simulink model "Power_windows"  (R2017b)
settings: Solver=VariableStepAuto  StartTime=0.0  StopTime=30  RelTol=1e-3
undefined symbols (not defined in the file): sigbuilder_block
libraries: simulink x1
settings Model: PauseTimes=10  SnapshotBufferSize=1  SnapshotInterval=1  Creator=ECoDe_user13  LastModifiedBy=ECoDe_user11
settings DebuggingCC: SignalInfNanChecking=error  UniqueDataStoreMsg=error  StrictBusMsg=ErrorOnBusTreatedAsVector
settings ConfigComp: CovEnable=on  RecordCoverage=on  CovMetricSettings=dcmwe  CovModelRefEnable=on

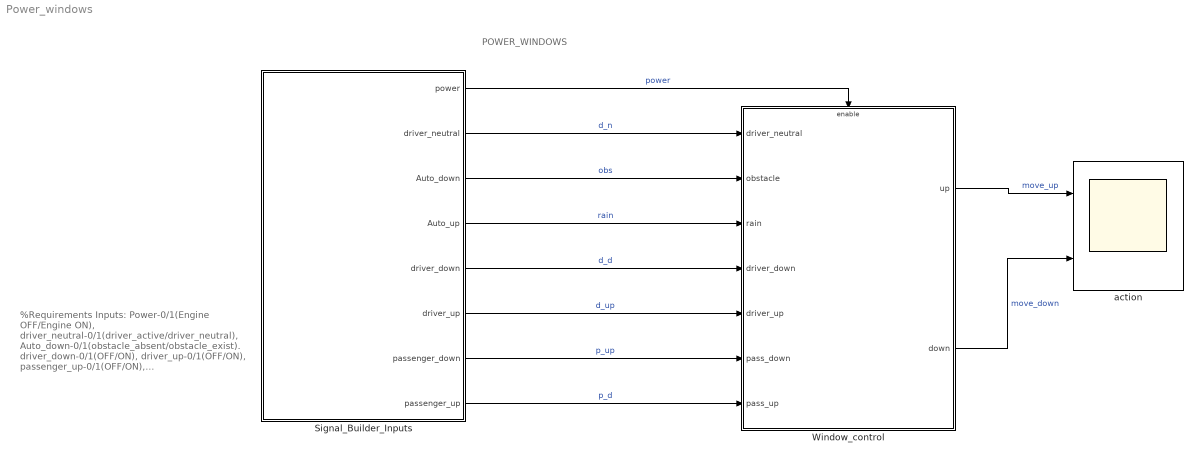
== system Power_windows ==
  note: POWER_WINDOWS
  note: %Requirements
      | Inputs:
      | Power-0/1(Engine OFF/Engine ON),
      | driver_neutral-0/1(driver_active/driver_neutral),
      | Auto_down-0/1(obstacle_absent/obstacle_exist).
      | driver_down-0/1(OFF/ON),
      | driver_up-0/1(OFF/ON),
      | passenger_up-0/1(OFF/ON),
      | passenger_down-0/1(OFF/ON),
      | Outputs:
      | Move_up-0/1(Either_neutral/UP),
      | Move_down-0/1(Either_neutral/Down.
  Signal_Builder_Inputs : Subsystem  Tag=STV Subsys  LoadFcn=sigbuilder_block('load',[3 150.75 550.5 369 ]);  StartFcn=sigbuilder_block('start');  StopFcn=sigbuilder_block('stop');  ClipboardFcn=sigbuilder_block('clipboard');  mask(Sigbuilder block){tuvar=[0:10]}
      mask help: Simulink:masks:SigbuilderBlock_MD
      mask init:
      | if ~strcmp(get_param(bdroot(gcbh),'SimulationStatus'),'stopped') tuvar = sigbuilder_block('maskInit'); end
      settings: CopyFcn=sigbuilder_block('copy');  DeleteFcn=sigbuilder_block('delete');  ModelCloseFcn=sigbuilder_block('modelClose');  PreSaveFcn=sigbuilder_block('preSave');  PauseFcn=sigbuilder_block('pause');  ContinueFcn=sigbuilder_block('continue');  NameChangeFcn=sigbuilder_block('namechange');  OpenFcn=sigbuilder_block('open',[3 150.75 550.5 369 ]);  CloseFcn=sigbuilder_block('close');
      mask Display: plot(0, 0, 100, 100,[2, 2, 32, 32, 2], [68, 8, 8, 68, 68],[32, 2], [38, 38], [32, 19, 2],[53, 60, 44], [32, 17, 17, 2],[16, 16, 31, 31]);txt = getActiveGroup(gcbh);text(2, 100, txt,'verticalAlignment', 'top');
  Window_control : Subsystem
  action : Scope  NumInputPorts=2
  wires:
  Signal_Builder_Inputs/1(power) -> Window_control/Enable  "power"
  Signal_Builder_Inputs/3(Auto_down) -> Window_control/2(obstacle)  "obs"
  Signal_Builder_Inputs/4(Auto_up) -> Window_control/3(rain)  "rain"
  Signal_Builder_Inputs/5(driver_down) -> Window_control/4(driver_down)  "d_d"
  Signal_Builder_Inputs/6(driver_up) -> Window_control/5(driver_up)  "d_up"
  Signal_Builder_Inputs/7(passenger_down) -> Window_control/6(pass_down)  "p_up"
  Signal_Builder_Inputs/8(passenger_up) -> Window_control/7(pass_up)  "p_d"
  Window_control/1(up) -> action/1  "move_up"
  Window_control/2(down) -> action/2  "move_down"
  Signal_Builder_Inputs/2(driver_neutral) -> Window_control/1(driver_neutral)  "d_n"

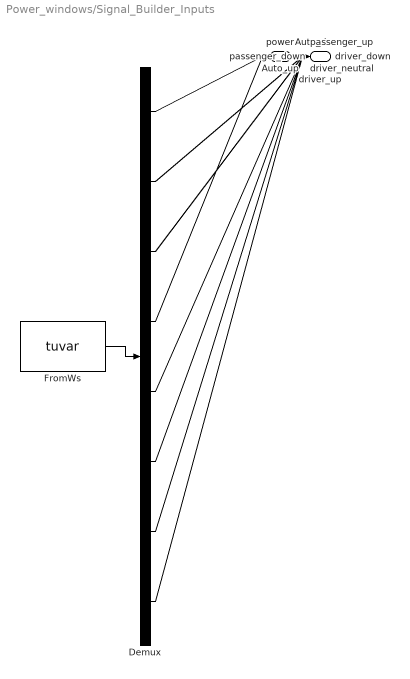
== system Power_windows/Signal_Builder_Inputs ==
  Demux : Demux  Tag=STV Demux  Outputs=8
  FromWs : FromWorkspace  Tag=STV FromWs  VariableName=tuvar  SampleTime=0
      SigBuilderData=|
      | common.afterFinalStr = 'Extrapolate'
      | common.sampleTime = 0
      | dataSet.timeRange = [0 28]
      | dataSet.name = 'Inputs'
      | sbobj.Name = 'Signal Builder'
      | sbobj.Groups.Name = 'Inputs'
      | sbobj.Groups.Signals(1).Name = 'power'
      | sbobj.Groups.Signals(1).XData = [0 1 2 3 4 5 6 7 8 9 10 11 12 13 14 15 16 17 18 19 20 20 21 21 22 22 23 24 25 26 26 27 28]
      | sbobj.Groups.Signals(1).YData = [1 1 1 1 1 1 1 1 1 1 1 1 1 1 1 1 1 1 1 1 1 0 0 1 1 0 0 0 0 0 1 1 1]
      | sbobj.Groups.Signals(2).Name = 'driver_neutral'
      | sbobj.Groups.Signals(2).XData = [0 1 1 2 3 3 4 5 5 6 6 7 8 8 9 10 10 11 11 12 13 13 14 15 15 16 16 17 18 18 19 20 21 22 22 23 23 24 25 26 27 28]
      | sbobj.Groups.Signals(2).YData = [0 0 1 1 1 0 0 0 1 1 0 0 0 1 1 1 0 0 1 1 1 0 0 0 1 1 0 0 0 1 1 1 1 1 0 0 1 1 1 1 1 1]
      | sbobj.Groups.Signals(3).Name = 'Auto_down'
      | sbobj.Groups.Signals(3).XData = [0 1 2 3 4 5 5 6 6 7 8 9 10 11 12 13 14 15 15 16 16 17 18 19 20 21 21 22 22 23 24 25 26 26 27 28]
      | sbobj.Groups.Signals(3).YData = [0 0 0 0 0 0 1 1 0 0 0 0 0 0 0 0 0 0 1 1 0 0 0 0 0 0 1 1 0 0 0 0 0 1 1 1]
      | sbobj.Groups.Signals(4).Name = 'Auto_up'
      | sbobj.Groups.Signals(4).XData = [0 1 2 2 3 3 4 5 6 7 7 8 8 9 9 10 10 11 12 12 13 13 14 15 16 17 17 18 18 19 19 20 20 21 21 22 23 23 24 24 25 25 26 26 27 28]
      | sbobj.Groups.Signals(4).YData = [0 0 0 1 1 0 0 0 0 0 1 1 0 0 1 1 0 0 0 1 1 0 0 0 0 0 1 1 0 0 1 1 0 0 1 1 1 0 0 1 1 0 0 1 1 1]
      | sbobj.Groups.Signals(5).Name = 'driver_down'
      | sbobj.Groups.Signals(5).XData = [0 1 1 2 3 3 4 4 5 6 6 7 8 8 9 10 10 11 11 12 13 13 14 14 15 16 16 17 18 18 19 20 21 22 22 23 23 24 25 25 26 27 28]
      | sbobj.Groups.Signals(5).YData = [1 1 0 0 0 1 1 0 0 0 1 1 1 0 0 0 1 1 0 0 0 1 1 0 0 0 1 1 1 0 0 0 0 0 1 1 0 0 0 1 1 1 1]
      | sbobj.Groups.Signals(6).Name = 'driver_up'
      | sbobj.Groups.Signals(6).XData = [0 1 2 3 4 4 5 5 6 7 8 9 10 11 12 13 14 14 15 15 16 17 18 19 20 21 21 22 22 23 24 25 26 26 27 27 28]
      | sbobj.Groups.Signals(6).YData = [0 0 0 0 0 1 1 0 0 0 0 0 0 0 0 0 0 1 1 0 0 0 0 0 0 0 1 1 0 0 0 0 0 1 1 0 0]
      | sbobj.Groups.Signals(7).Name = 'passenger_down'
      | sbobj.Groups.Signals(7).XData = [0 1 2 3 4 4 5 5 6 7 7 8 9 10 10 11 11 12 12 13 14 14 15 15 16 17 17 18 19 20 20 21 21 22 23 24 25 25 26 26 27 28]
      | sbobj.Groups.Signals(7).YData = [0 0 0 0 0 1 1 0 0 0 1 1 1 1 0 0 1 1 0 0 0 1 1 0 0 0 1 1 1 1 0 0 1 1 1 1 1 0 0 1 1 1]
      | sbobj.Groups.Signals(8).Name = 'passenger_up'
      | sbobj.Groups.Signals(8).XData = [0 1 1 2 2 3 3 4 4 5 5 6 7 7 8 9 10 11 12 13 13 14 14 15 15 16 17 17 18 19 20 21 21 22 22 23 24 25 26 26 27 27 28]
      | sbobj.Groups.Signals(8).YData = [0 0 1 1 0 0 1 1 0 0 1 1 1 0 0 0 0 0 0 0 1 1 0 0 1 1 1 0 0 0 0 0 1 1 0 0 0 0 0 1 1 0 0]
      | sbobj.Groups.TimeRange = [0 28]
  power : Outport  Tag=STV Outport
  driver_neutral : Outport  Tag=STV Outport  Port=2
  Auto_down : Outport  Tag=STV Outport  Port=3
  Auto_up : Outport  Tag=STV Outport  Port=4
  driver_down : Outport  Tag=STV Outport  Port=5
  driver_up : Outport  Tag=STV Outport  Port=6
  passenger_down : Outport  Tag=STV Outport  Port=7
  passenger_up : Outport  Tag=STV Outport  Port=8
  wires:
  FromWs/1 -> Demux/1
  Demux/1 -> power/1
  Demux/2 -> driver_neutral/1
  Demux/3 -> Auto_down/1
  Demux/4 -> Auto_up/1
  Demux/5 -> driver_down/1
  Demux/6 -> driver_up/1
  Demux/7 -> passenger_down/1
  Demux/8 -> passenger_up/1

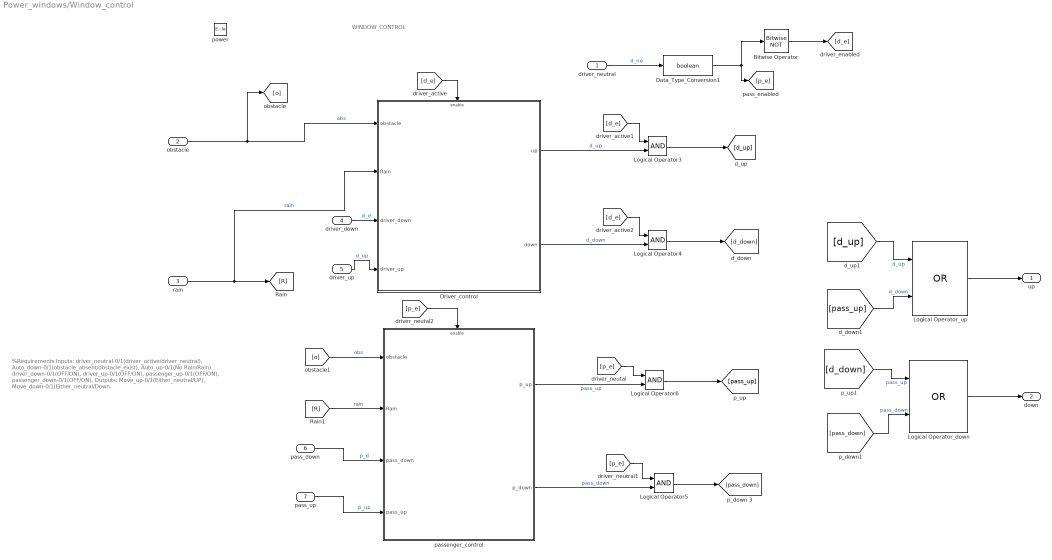
== system Power_windows/Window_control ==
  note: %Requirements
      | Inputs:
      | driver_neutral-0/1(driver_active/driver_neutral),
      | Auto_down-0/1(obstacle_absent/obstacle_exist),
      | Auto_up-0/1(No Rain/Rain)
      | driver_down-0/1(OFF/ON),
      | driver_up-0/1(OFF/ON),
      | passenger_up-0/1(OFF/ON),
      | passenger_down-0/1(OFF/ON),
      | Outputs:
      | Move_up-0/1(Either_neutral/UP),
      | Move_down-0/1(Either_neutral/Down.
  note: WINDOW_CONTROL
  driver_neutral : Inport
  obstacle : Inport  Port=2
  rain : Inport  Port=3
  driver_down : Inport  Port=4
  driver_up : Inport  Port=5
  pass_down : Inport  Port=6
  pass_up : Inport  Port=7
  power : EnablePort
  Bitwise Operator : simulink/Logic and Bit Operations/Bitwise Operator  logicop=NOT  UseBitMask=off  BitMask=bin2dec('11011001')  BitMaskRealWorld=Stored Integer
  Data_Type_Conversion1 : DataTypeConversion  OutDataTypeStr=boolean
  Driver_control : Subsystem
  Logical Operator{3..6} (4 alike) : Logic  AllPortsSameDT=off  OutDataTypeStr=boolean
  Logical Operator_down : Logic  Operator=OR  AllPortsSameDT=off  OutDataTypeStr=boolean
  "Logical Operator_up " : Logic  Operator=OR  AllPortsSameDT=off  OutDataTypeStr=boolean
  passenger_control : Subsystem
  up : Outport
  down : Outport  Port=2
  wires:
  Logical Operator_down/1 -> down/1
  "Logical Operator_up "/1 -> up/1
  Driver_control/1(up) -> Logical Operator3/2  "d_up"
  driver_up/1 -> Driver_control/4(driver_up)  "d_up"
  driver_down/1 -> Driver_control/3(driver_down)  "d_d"
  rain/1 -> [R], Driver_control/2(Rain)  "rain"
  obstacle/1 -> [o], Driver_control/1(obstacle)  "obs"
  pass_down/1 -> passenger_control/3(pass_down)  "p_d"
  pass_up/1 -> passenger_control/4(pass_up)  "p_up"
  Driver_control/2(down) -> Logical Operator4/2  "d_down"
  driver_neutral/1 -> Data_Type_Conversion1/1  "d_ne"
  Data_Type_Conversion1/1 -> [p_e], Bitwise Operator/1
  passenger_control/1(p_up) -> Logical Operator6/2  "pass_up"
  passenger_control/2(p_down) -> Logical Operator5/2  "pass_down"
  [p_e] -> passenger_control/Enable
  [p_e] -> Logical Operator6/1
  [p_e] -> Logical Operator5/1
  Bitwise Operator/1 -> [d_e]
  [d_e] -> Driver_control/Enable
  [d_e] -> Logical Operator3/1
  [d_e] -> Logical Operator4/1
  Logical Operator3/1 -> [d_up]
  Logical Operator6/1 -> [pass_up]
  Logical Operator5/1 -> [pass_down]
  Logical Operator4/1 -> [d_down]
  [d_up] -> "Logical Operator_up "/1  "d_up"
  [pass_up] -> "Logical Operator_up "/2  "d_down"
  [d_down] -> Logical Operator_down/1  "pass_up"
  [pass_down] -> Logical Operator_down/2  "pass_down"
  [o] -> passenger_control/1(obstacle)  "obs"
  [R] -> passenger_control/2(Rain)  "rain"

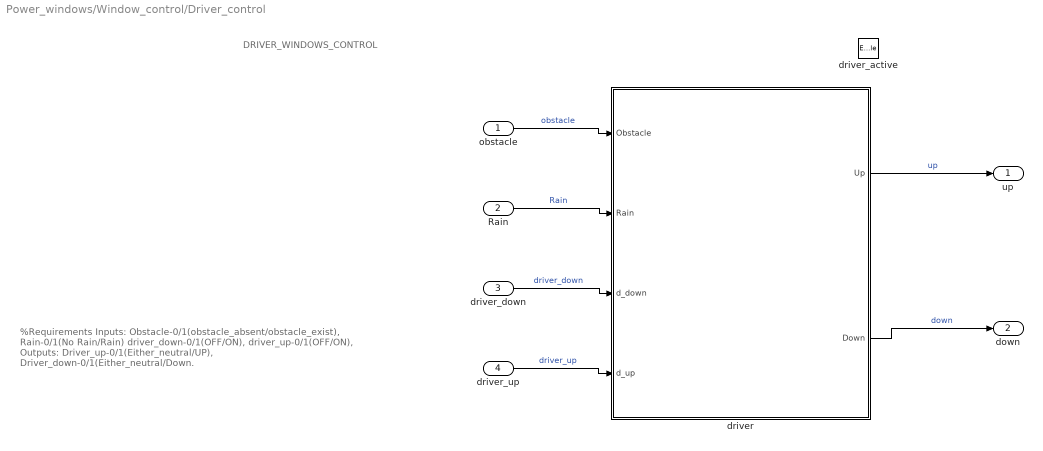
== system Power_windows/Window_control/Driver_control ==
  note: %Requirements
      | Inputs:
      | Obstacle-0/1(obstacle_absent/obstacle_exist),
      | Rain-0/1(No Rain/Rain)
      | driver_down-0/1(OFF/ON),
      | driver_up-0/1(OFF/ON),
      |
      | Outputs:
      | Driver_up-0/1(Either_neutral/UP),
      | Driver_down-0/1(Either_neutral/Down.
  note: DRIVER_WINDOWS_CONTROL
  obstacle : Inport
  Rain : Inport  Port=2
  driver_down : Inport  Port=3
  driver_up : Inport  Port=4
  driver_active : EnablePort
  driver : Stateflow chart  TreatAsAtomicUnit=on
  up : Outport
  down : Outport  Port=2
  wires:
  driver_up/1 -> driver/4(d_up)  "driver_up"
  driver/1(Up) -> up/1  "up"
  driver/2(Down) -> down/1  "down"
  obstacle/1 -> driver/1(Obstacle)  "obstacle"
  Rain/1 -> driver/2(Rain)  "Rain"
  driver_down/1 -> driver/3(d_down)  "driver_down"

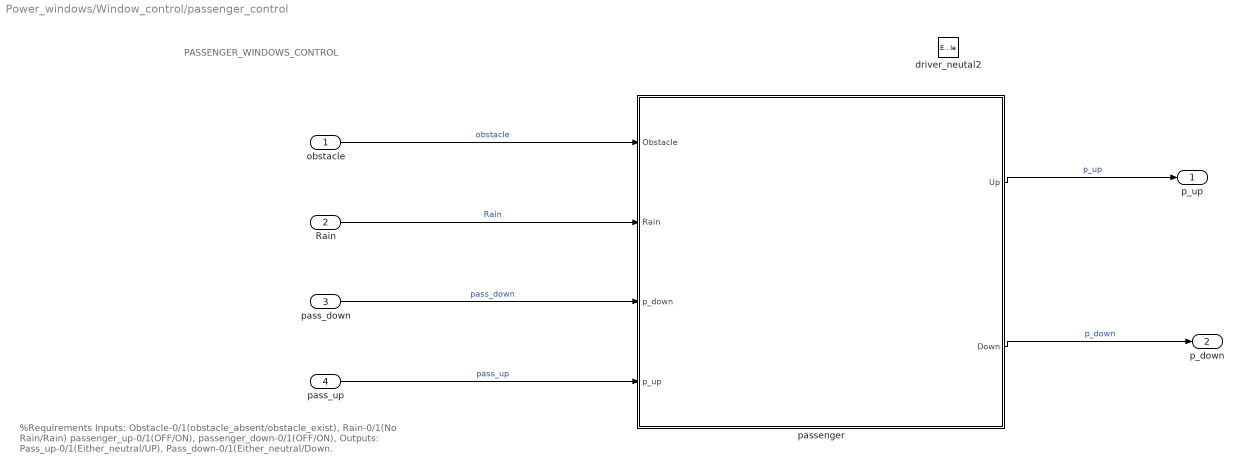
== system Power_windows/Window_control/passenger_control ==
  note: %Requirements
      | Inputs:
      | Obstacle-0/1(obstacle_absent/obstacle_exist),
      | Rain-0/1(No Rain/Rain)
      | passenger_up-0/1(OFF/ON),
      | passenger_down-0/1(OFF/ON),
      | Outputs:
      | Pass_up-0/1(Either_neutral/UP),
      | Pass_down-0/1(Either_neutral/Down.
  note: PASSENGER_WINDOWS_CONTROL
  obstacle : Inport
  Rain : Inport  Port=2
  pass_down : Inport  Port=3
  pass_up : Inport  Port=4
  driver_neutal2 : EnablePort
  passenger : Stateflow chart  TreatAsAtomicUnit=on
  p_up : Outport
  p_down : Outport  Port=2
  wires:
  pass_up/1 -> passenger/4(p_up)  "pass_up"
  pass_down/1 -> passenger/3(p_down)  "pass_down"
  Rain/1 -> passenger/2(Rain)  "Rain"
  passenger/2(Down) -> p_down/1  "p_down"
  passenger/1(Up) -> p_up/1  "p_up"
  obstacle/1 -> passenger/1(Obstacle)  "obstacle"

== stateflow chart Power_windows/Window_control/Driver_control/driver ==
  state NormalState
    state Neutral
      entry:
      Up=0;
      Down=0;
    state Up
      entry:
      Up=1;
      Down=0;
    state Down
      entry:
      Up=0;
      Down=1;
    (default) -> Neutral
    Neutral -> Down [order 1] : [d_up==0&&d_down==1]
    Up -> Neutral [order 2] : [[d_up==0&&d_down==0]]
    Down -> Neutral [order 2] : [d_up==0&&d_down==0]
    Neutral -> Up [order 2] : [d_up==1&&d_down==0]
    Down -> Up [order 1] : [d_up==1&&d_down==0]
    Up -> Down [order 1] : [d_up==0&&d_down==1]
  state Obstacle
    entry:
    Up=0;
    Down=1;
  state Rain
    entry:
    Up=1;
    Down=0;
  (default) -> NormalState
  Rain -> Neutral : [Rain==0]
  Obstacle -> Neutral : [Obstacle==0]
  NormalState -> Obstacle [order 1] : [Obstacle==1]
  NormalState -> Rain [order 2] : [Rain==1]
  data: Obstacle input; Rain input; Up output; Down output; d_down input; d_up input

== stateflow chart Power_windows/Window_control/passenger_control/passenger ==
  state NormalState
    state Neutral
      entry:
      Up=0;
      Down=0;
    state Up
      entry:
      Up=1;
      Down=0;
    state Down
      entry:
      Up=0;
      Down=1;
    (default) -> Neutral
    Neutral -> Down [order 1] : [p_up==0&&p_down==1]
    Up -> Neutral [order 2] : [[p_up==0&&p_down==0]]
    Down -> Neutral [order 2] : [p_up==0&&p_down==0]
    Neutral -> Up [order 2] : [p_up==1&&p_down==0]
    Down -> Up [order 1] : [p_up==1&&p_down==0]
    Up -> Down [order 1] : [p_up==0&&p_down==1]
  state Obstacle
    entry:
    Up=0;
    Down=1;
  state Rain
    entry:
    Up=1;
    Down=0;
  (default) -> NormalState
  Rain -> Neutral : [Rain==0]
  Obstacle -> Neutral : [Obstacle==0]
  NormalState -> Obstacle [order 1] : [Obstacle==1]
  NormalState -> Rain [order 2] : [Rain==1]
  data: Obstacle input; Up output; Down output; Rain input; p_down input; p_up input
